simulink model "AutomaticPrintingKiosk_Matlab"  (R2024b)
settings: Solver=VariableStepAuto  StartTime=0.0  StopTime=10.0  RelTol=1e-3
undefined symbols (not defined in the file or in its folder): Rec, SDTV
libraries: visionconversions x2, visionanalysis x1
settings Model: Creator=PARTHA PRATIM ROY  LastModifiedBy=hp

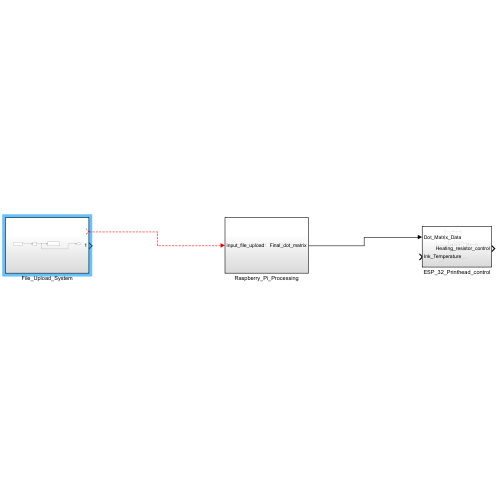
[thumbnail: Simulink's stored preview of the top-level diagram]
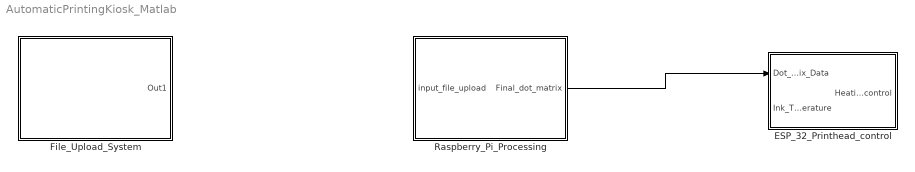
== system AutomaticPrintingKiosk_Matlab ==
  ESP_32_Printhead_control : Subsystem
  File_Upload_System : Subsystem
  Raspberry_Pi_Processing : Subsystem
  wires:
  Raspberry_Pi_Processing/1(Final_dot_matrix) -> ESP_32_Printhead_control/1(Dot_Matrix_Data)
  ? -> Raspberry_Pi_Processing/1(input_file_upload)

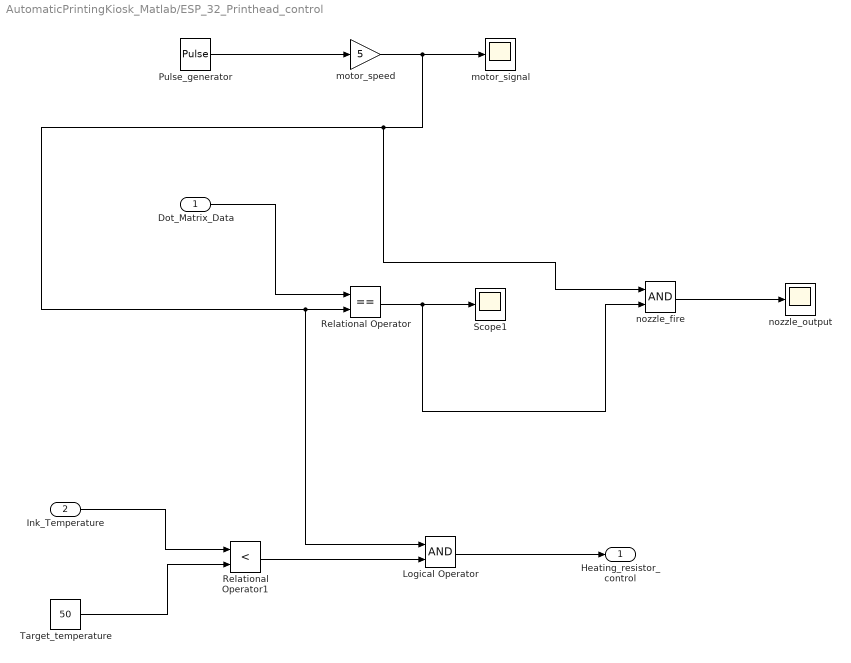
== system AutomaticPrintingKiosk_Matlab/ESP_32_Printhead_control ==
  Dot_Matrix_Data : Inport
  Ink_Temperature : Inport  Port=2
  Logical Operator : Logic  AllPortsSameDT=off  OutDataTypeStr=boolean
  Pulse_generator : DiscretePulseGenerator  PulseType=Time based  Period=0.02  PulseWidth=50
  Relational Operator : RelationalOperator  Operator===  OutDataTypeStr=boolean  RndMeth=Simplest  InputSameDT=off
  Relational Operator1 : RelationalOperator  Operator=<  OutDataTypeStr=boolean  RndMeth=Simplest  InputSameDT=off
  Scope1 : Scope
  Target_temperature : Constant  Value=50
  motor_signal : Scope
  motor_speed : Gain  Gain=5
  nozzle_fire : Logic  AllPortsSameDT=off  OutDataTypeStr=boolean
  nozzle_output : Scope
  Heating_resistor_control : Outport
  wires:
  Pulse_generator/1 -> motor_speed/1
  Dot_Matrix_Data/1 -> Relational Operator/1
  Relational Operator/1 -> nozzle_fire/2, Scope1/1
  motor_speed/1 -> nozzle_fire/1, Logical Operator/1, Relational Operator/2, motor_signal/1
  nozzle_fire/1 -> nozzle_output/1
  Ink_Temperature/1 -> Relational Operator1/1
  Target_temperature/1 -> Relational Operator1/2
  Relational Operator1/1 -> Logical Operator/2
  Logical Operator/1 -> Heating_resistor_control/1

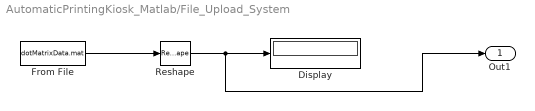
== system AutomaticPrintingKiosk_Matlab/File_Upload_System ==
  Display : Display
  From File : FromFile  FileName=dotMatrixData.mat  SampleTime=0
  Reshape : Reshape
  Out1 : Outport
  wires:
  From File/1 -> Reshape/1
  Reshape/1 -> Out1/1, Display/1

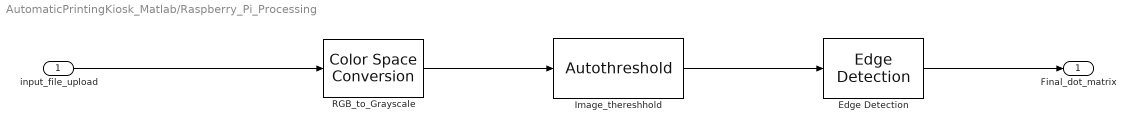
== system AutomaticPrintingKiosk_Matlab/Raspberry_Pi_Processing ==
  input_file_upload : Inport
  Edge Detection : visionanalysis/Edge Detection  method=Canny  outputType=Binary image  userDefinedThreshold=off  thresholdSource=Input port  threshold=20  thresholdTuning=4  edgeThinning=off  threshold_canny=[0.25 0.60]  autoPercent=70  sigma=1  roundingMode=Floor  overflowMode=off  prodOutputMode=Binary point scaling  prodOutputWordLength=32  prodOutputFracLength=8
  Image_thereshhold : visionconversions/Autothreshold  operator=>  threshOut=off  effMetricOut=off  userDefinedRange=off  umin=0  umax=255  outOfRngOpt=Ignore  scaleThreshold=off  scaleFactor=1  roundingMode=Floor  overflowMode=off  P1Mode=Specify word length  P1WordLength=32  P1FracLength=30  P2Mode=Specify word length  P2WordLength=32  P2FracLength=22  P3Mode=Specify word length  P3WordLength=32  P3FracLength=14  P4Mode=Binary point scaling  P4WordLength=32  P4FracLength=15  Q1Mode=Specify word length  Q1WordLength=32  Q1FracLength=16  EMMode=Specify word length  EMWordLength=16  EMFracLength=14
  RGB_to_Grayscale : visionconversions/Color Space  Conversion  conversion=Obsolete  conversionActive=R'G'B' to intensity  wp_str=D65  rec=Rec. 601 (SDTV)  sys=1125/60/2:1  imagePorts=One multidimensional signal
  Final_dot_matrix : Outport
  wires:
  RGB_to_Grayscale/1 -> Image_thereshhold/1
  Image_thereshhold/1 -> Edge Detection/1
  Edge Detection/1 -> Final_dot_matrix/1
  input_file_upload/1 -> RGB_to_Grayscale/1
